simulink model "soc_dvbs2_fpga"  (R2025b)
settings: Solver=FixedStepDiscrete  StartTime=0.0  StopTime=0  RelTol=1e-3
InitFcn:
  | soc_dvbs2_init;
values from neighbouring files (symbols this model uses):
  Rsym = 4e6    (= 4000000)    [soc_dvbs2_init.m]
  soc_dvbs2_txPacketBits = [1 1 0 1 0 1 1 1 0 1 1 1 ... (2972 elements, 2972x1)]    [soc_dvbs2_txPacketBits.mat]
  syncWord = (dec2bin(hex2dec('AC')) - '0').'    [soc_dvbs2_init.m]
  txDataOut = txobj(frameBits(:))    [soc_dvbs2_init.m]
  txFiltCoeff = txobj.pTxFilterCoeff    [soc_dvbs2_init.m]
undefined symbols (not defined in the file or in its folder): Add, coefficientsLog, coefficientsSqrt1, coefficientsSqrt2, dataBits, designMultirateFIR, noisePow, NumBits1, NumBits2, seedsURNG1, seedsURNG2, Shift, Slope1, Slope2, soc_dvbs2_designFIRFilter, txDataOutS1, txDataOutS10, txDataOutS12, txDataOutS13, txDataOutS14, txDataOutS15, txDataOutS16, txDataOutS18, txDataOutS19, txDataOutS2, txDataOutS20, txDataOutS21, txDataOutS22, txDataOutS24, txDataOutS25, txDataOutS26, txDataOutS27, txDataOutS3, txDataOutS4, txDataOutS5, txDataOutS6, txDataOutS7, txDataOutS8, txDataOutS9
libraries: simulink x214, hdlsllib x211, dspsigops x22, dsphdlfiltering2 x8, dsphdlsigops2 x5, commseqgen3 x5, dsphdlmathfun2 x3, hwlogicconnlib x2, whdledac x2, commhdlcrc x2, whdlutilities x1, whdlmod x1
(part 3 of 12)

== system soc_dvbs2_fpga/DVBS2/DVBS2 TxRx/DVB-S2 HDL Receiver/Stream Recovery/BB Header CRC Check ==
  dstartIn : Inport
  dValidIn : Inport  Port=2
  bitsIn : Inport  Port=3
  hstartIn : Inport  Port=4
  hendIn : Inport  Port=5
  hvalidIn : Inport  Port=6
  Delay{,1..3,8..13,15} (11 alike) : Delay  DelayLength=1
  Delay4 : Delay  DelayLength=26
  Delay6 : Delay  DelayLength=26
  Delay7 : Delay  DelayLength=26
  Discard CRC failed Frame : Subsystem
  General CRC Syndrome Detector HDL Optimized : commhdlcrc/General CRC Syndrome Detector HDL Optimized  Polynomial=[1 1 1 0 1 0 1 0 1]  InitialState=0  DirectMethod=off  ReflectInput=off  ReflectCRCChecksum=off  FinalXORValue=0  SimulateUsing=Code generation
  dstartOut : Outport
  dvalidIn : Outport  Port=2
  dbitsOut : Outport  Port=3
  hbitsOut : Outport  Port=4
  hstartOut : Outport  Port=5
  hendOut : Outport  Port=6
  hvalidOut : Outport  Port=7
  herrorOut : Outport  Port=8
  wires:
  Delay15/1 -> Delay4/1
  dValidIn/1 -> Delay13/1
  Delay12/1 -> General CRC Syndrome Detector HDL Optimized/4
  Delay11/1 -> General CRC Syndrome Detector HDL Optimized/3
  Delay10/1 -> General CRC Syndrome Detector HDL Optimized/2
  Delay9/1 -> General CRC Syndrome Detector HDL Optimized/1, Delay7/1
  Discard CRC failed Frame/3(bitsOut) -> dbitsOut/1
  Discard CRC failed Frame/2(validOut) -> dvalidIn/1
  Discard CRC failed Frame/1(startOut) -> dstartOut/1
  Delay7/1 -> Discard CRC failed Frame/3(bitsIn)
  Delay6/1 -> Discard CRC failed Frame/2(validIn)
  Delay4/1 -> Discard CRC failed Frame/1(startIn)
  Delay8/1 -> hbitsOut/1
  Delay3/1 -> hstartOut/1
  Delay2/1 -> hendOut/1
  Delay1/1 -> hvalidOut/1
  Delay/1 -> herrorOut/1
  General CRC Syndrome Detector HDL Optimized/5 -> Delay/1, Discard CRC failed Frame/4(err)
  General CRC Syndrome Detector HDL Optimized/4 -> Delay1/1
  General CRC Syndrome Detector HDL Optimized/1 -> Delay8/1
  hvalidIn/1 -> Delay12/1
  hstartIn/1 -> Delay10/1
  bitsIn/1 -> Delay9/1
  General CRC Syndrome Detector HDL Optimized/3 -> Delay2/1, Discard CRC failed Frame/5(errorValid)
  dstartIn/1 -> Delay15/1
  Delay13/1 -> Delay6/1
  hendIn/1 -> Delay11/1
  General CRC Syndrome Detector HDL Optimized/2 -> Delay3/1

== system soc_dvbs2_fpga/DVBS2/DVBS2 TxRx/DVB-S2 HDL Receiver/Synchronizer and PL Header Decoder/Enable MODCOD  ==
  note: force MODCOD to 0 until synchronization is done
  modcod : Inport
  enb : Inport  Port=2
  Constant : Constant  Value=0  OutDataTypeStr=Inherit: Inherit via back propagation  SampleTime=-1
  Constant1 : Constant  Value=modcodToZero  OutDataTypeStr=boolean  SampleTime=-1
  Switch : Switch  Criteria=u2 ~= 0  SaturateOnIntegerOverflow=off  InputSameDT=off
  Switch1 : Switch  Criteria=u2 ~= 0  SaturateOnIntegerOverflow=off  InputSameDT=off
  modcodOut : Outport
  wires:
  modcod/1 -> Switch1/3, Switch/1
  Switch/1 -> Switch1/1
  enb/1 -> Switch/2
  Constant/1 -> Switch/3
  Constant1/1 -> Switch1/2
  Switch1/1 -> modcodOut/1

== system soc_dvbs2_fpga/DVBS2/DVBS2 TxRx/DVB-S2 HDL Receiver/Synchronizer and PL Header Decoder/Fine Phase Synchronizer ==
  dataIn : Inport
  validIn : Inport  Port=2
  endOfPLSCIn : Inport  Port=3
  mod : Inport  Port=4
  En : Inport  Port=5
  rst : Inport  Port=6
  Data Type Conversion : DataTypeConversion  OutDataTypeStr=fixdt(1,18,14)  SaturateOnIntegerOverflow=off  RndMeth=Floor
  Data Type Conversion1 : DataTypeConversion  OutDataTypeStr=fixdt(1,22,14)  SaturateOnIntegerOverflow=off  RndMeth=Floor
  Delay{1..4,12..14} (7 alike) : Delay  DelayLength=1
  Delay{5..11,15..16} (9 alike) : Delay
  Direct Digital Synthesis : Subsystem
  Loop Filter : Subsystem
  Math Function : Math  Operator=conj
  Phase Error Detector : Subsystem
  Power Q and Beta Offset Rotation : Subsystem
  Product : Product
  dataOut : Outport
  validOut : Outport  Port=2
  endOfPLSC : Outport  Port=3
  wires:
  Loop Filter/2(rstOut) -> Direct Digital Synthesis/2(rst)
  rst/1 -> Loop Filter/3(rst)
  En/1 -> Loop Filter/2(En)
  Data Type Conversion1/1 -> Delay12/1, Delay15/1
  Power Q and Beta Offset Rotation/1(dataOut) -> Phase Error Detector/1(dataIn)
  Loop Filter/1(v) -> Direct Digital Synthesis/1(v)
  Data Type Conversion/1 -> dataOut/1
  Delay16/1 -> Power Q and Beta Offset Rotation/2(mod)
  Delay15/1 -> Power Q and Beta Offset Rotation/1(dataIn)
  Delay14/1 -> endOfPLSC/1
  Delay13/1 -> validOut/1
  Delay12/1 -> Data Type Conversion/1
  Delay11/1 -> Delay14/1
  Delay10/1 -> Delay13/1
  Delay9/1 -> Delay11/1
  Delay8/1 -> Delay10/1
  Delay7/1 -> Data Type Conversion1/1
  Delay6/1 -> Product/2
  Delay5/1 -> Product/1
  endOfPLSCIn/1 -> Delay3/1
  validIn/1 -> Delay2/1
  Delay4/1 -> Delay5/1
  Delay1/1 -> Delay16/1
  Math Function/1 -> Delay6/1
  Direct Digital Synthesis/1(xph) -> Math Function/1
  Phase Error Detector/1(e) -> Loop Filter/1(e)
  mod/1 -> Delay1/1
  dataIn/1 -> Delay4/1
  Delay3/1 -> Delay9/1
  Product/1 -> Delay7/1
  Delay2/1 -> Delay8/1

== system soc_dvbs2_fpga/DVBS2/DVBS2 TxRx/DVB-S2 HDL Receiver/Synchronizer and PL Header Decoder/PL Header Recovery ==
  dataIn : Inport
  validIn : Inport  Port=2
  endOfSOF : Inport  Port=3
  hasPilots : Inport  Port=4
  Bus Creator : BusCreator  Inputs=2
  Delay{,1..3,5,11..20} (15 alike) : Delay  DelayLength=1
  Delay10 : Delay  DelayLength=46
  Delay4 : Delay  DelayLength=3
  Delay6 : Delay  DelayLength=3
  Delay7 : Delay  DelayLength=3
  Delay8 : Delay  DelayLength=46
  Delay9 : Delay  DelayLength=46
  No HDL : Subsystem
  No HDL1 : Subsystem
      settings: PortSchema="{\"entries\":[{\"content\":{\"sides\":[{\"content\":{\"connectorIds\":[\"In1\"]},\"type\":\"ConnectorPlacement.EquallySpacedRectSide\",\"uuid\":\"e49ce245-8ab6-4c67-8264-d94e0436676a\"},{\"content\":{\"connectorIds\":[\"In2\"],\"side\":\"RIGHT\"},\"type\":\"ConnectorPlacement.EquallySpacedRectSide\",\"uuid\":\"e18f2063-2732-4c7b-85c5-c61d406b5847\"},{\"content\":{\"connectorIds\":[],\"side\":\"TOP\"},\"type\":\"ConnectorPlacement.EquallySpacedRectSide\",\"uuid\":\"5432424d-e7f9-486b-a8e9-0d688bdbd9bb\"}]},\"type\":\"ConnectorPlacement.EquallySpacedConnector\",\"uuid\":\"00f6af48-98de-42b3-a1ba-3135a9ec94ea\"}],\"packageUris\":[\"http://schema.mathworks.com/mf0/Connector/R2020b\"],\"version\":\"1.0\"}"
  PL Frame Demultiplexer : Subsystem
  PL Header Decoder : Subsystem
  Unit Delay Enabled Synchronous : hdlsllib/Discrete/Unit Delay Enabled Synchronous  InitialCondition=0.0  SampleTime=-1
  Unit Delay Enabled Synchronous1 : hdlsllib/Discrete/Unit Delay Enabled Synchronous  InitialCondition=0.0  SampleTime=-1
  Unit Delay Enabled Synchronous2 : hdlsllib/Discrete/Unit Delay Enabled Synchronous  InitialCondition=0.0  SampleTime=-1
  PLSCDiag : Outport  VectorParamsAs1DForOutWhenUnconnected=off
  dataOut : Outport  Port=2  VectorParamsAs1DForOutWhenUnconnected=off
  validOut : Outport  Port=3  VectorParamsAs1DForOutWhenUnconnected=off
  endOfPLSC : Outport  Port=4  VectorParamsAs1DForOutWhenUnconnected=off
  modcod : Outport  Port=5  VectorParamsAs1DForOutWhenUnconnected=off
  FEC : Outport  Port=6  VectorParamsAs1DForOutWhenUnconnected=off
  wires:
  Unit Delay Enabled Synchronous2/1 -> FEC/1
  Unit Delay Enabled Synchronous/1 -> modcod/1
  Delay20/1 -> endOfPLSC/1
  Delay19/1 -> validOut/1
  Delay16/1 -> dataOut/1
  Bus Creator/1 -> PLSCDiag/1
  Delay18/1 -> No HDL1/2(endOfPLSc), Delay20/1, Unit Delay Enabled Synchronous/2, Unit Delay Enabled Synchronous2/2
  Delay17/1 -> Delay19/1
  Delay15/1 -> Unit Delay Enabled Synchronous2/1
  Delay14/1 -> Unit Delay Enabled Synchronous/1
  Delay13/1 -> Delay16/1
  Delay12/1 -> Delay13/1
  Delay11/1 -> Delay17/1
  Delay/1 -> Delay18/1
  Delay10/1 -> Delay12/1
  Delay9/1 -> Delay/1
  Delay8/1 -> Delay11/1
  Delay7/1 -> PL Header Decoder/3(endOfSOF)
  Delay6/1 -> PL Header Decoder/2(hasPilots)
  Delay4/1 -> Bus Creator/1, Delay10/1, PL Header Decoder/1(dataIn)  "PLSCSymb"
  Delay3/1 -> PL Frame Demultiplexer/2(validIn), No HDL1/1(valid)
  Delay2/1 -> Delay7/1, PL Frame Demultiplexer/1(endOfSOFIn), Unit Delay Enabled Synchronous1/2
  Delay1/1 -> Unit Delay Enabled Synchronous1/1
  Delay5/1 -> Delay4/1
  PL Frame Demultiplexer/3(endOfPLSC) -> Delay9/1
  PL Frame Demultiplexer/2(dValid) -> Delay8/1
  validIn/1 -> Delay3/1
  PL Frame Demultiplexer/1(hValid) -> PL Header Decoder/4(validIn), Bus Creator/2  "PLSCSymbValid"
  PL Header Decoder/2(FECFrame) -> Delay15/1
  Unit Delay Enabled Synchronous1/1 -> Delay6/1
  hasPilots/1 -> No HDL/1(has Pilots), Delay1/1
  endOfSOF/1 -> No HDL/Enable, Delay2/1
  PL Header Decoder/1(modcod) -> Delay14/1
  dataIn/1 -> Delay5/1

== system soc_dvbs2_fpga/DVBS2/DVBS2 TxRx/DVB-S2 HDL Receiver/Synchronizer and PL Header Decoder/Source Encoding ==
  modcod : Inport
  Delay1 : Delay  DelayLength=1
  Delay12 : Delay  DelayLength=1
  MATLAB Function : MATLAB Function  TreatAsAtomicUnit=on
  Terminator : Terminator
  mod : Outport
  wires:
  Delay1/1 -> mod/1
  Delay12/1 -> MATLAB Function/1(In)
  MATLAB Function/2(isdummy) -> Terminator/1
  MATLAB Function/1(out) -> Delay1/1
  modcod/1 -> Delay12/1

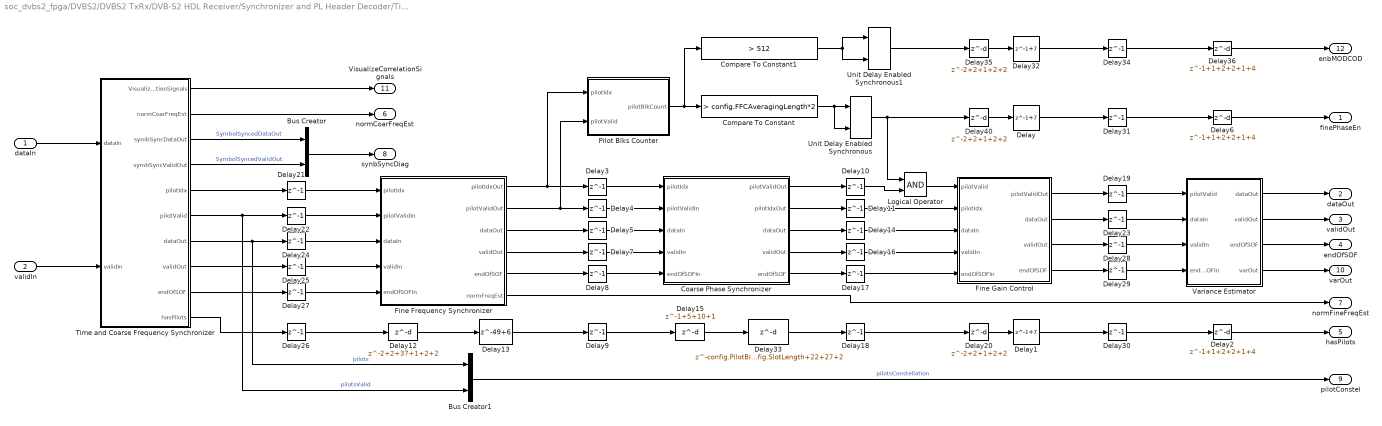
== system soc_dvbs2_fpga/DVBS2/DVBS2 TxRx/DVB-S2 HDL Receiver/Synchronizer and PL Header Decoder/Time Frequency and Coarse Phase Synchronizer ==
  dataIn : Inport
  validIn : Inport  Port=2
  Bus Creator : BusCreator  Inputs=2
  Bus Creator1 : BusCreator  Inputs=2
  Coarse Phase Synchronizer : Subsystem
  Compare To Constant : simulink/Logic and Bit Operations/Compare To Constant  relop=>  const=config.FFCAveragingLength*2  OutDataTypeStr=boolean
  Compare To Constant1 : simulink/Logic and Bit Operations/Compare To Constant  relop=>  const=512  OutDataTypeStr=boolean
  Delay : Delay  DelayLength=1+7
  Delay1 : Delay  DelayLength=1+7
  Delay{3..5,7..11,14,16..19,21..31,34} (25 alike) : Delay  DelayLength=1
  Delay12 : Delay  DelayLength=2+2+37+1+2+2
  Delay13 : Delay  DelayLength=49+6
  Delay15 : Delay  DelayLength=1+5+10+1
  Delay2 : Delay  DelayLength=1+1+2+2+1+4
  Delay20 : Delay  DelayLength=2+2+1+2+2
  Delay32 : Delay  DelayLength=1+7
  Delay33 : Delay  DelayLength=config.PilotBlkFreq*config.SlotLength+22+27+2
  Delay35 : Delay  DelayLength=2+2+1+2+2
  Delay36 : Delay  DelayLength=1+1+2+2+1+4
  Delay40 : Delay  DelayLength=2+2+1+2+2
  Delay6 : Delay  DelayLength=1+1+2+2+1+4
  Fine Frequency Synchronizer : Subsystem
  Fine Gain Control : Subsystem
  Logical Operator : Logic  AllPortsSameDT=off  OutDataTypeStr=boolean
  Pilot Blks Counter : Subsystem
  Time and Coarse Frequency Synchronizer : Subsystem
  Unit Delay Enabled Synchronous : hdlsllib/Discrete/Unit Delay Enabled Synchronous  InitialCondition=0.0  SampleTime=-1
  Unit Delay Enabled Synchronous1 : hdlsllib/Discrete/Unit Delay Enabled Synchronous  InitialCondition=0.0  SampleTime=-1
  Variance Estimator : Subsystem
  finePhaseEn : Outport
  dataOut : Outport  Port=2
  validOut : Outport  Port=3
  endOfSOF : Outport  Port=4
  hasPilots : Outport  Port=5
  normCoarFreqEst : Outport  Port=6
  normFineFreqEst : Outport  Port=7
  synbSyncDiag : Outport  Port=8
  pilotConstel : Outport  Port=9
  varOut : Outport  Port=10
  VisualizeCorrelationSignals : Outport  Port=11
  enbMODCOD : Outport  Port=12
  wires:
  Delay31/1 -> Delay6/1
  Delay30/1 -> Delay2/1
  Delay29/1 -> Variance Estimator/4(endOfSOFIn)
  Delay28/1 -> Variance Estimator/3(validIn)
  Delay23/1 -> Variance Estimator/2(dataIn)
  Delay19/1 -> Variance Estimator/1(pilotValid)
  Delay18/1 -> Delay20/1
  Delay17/1 -> Fine Gain Control/5(endOfSOFIn)
  Delay16/1 -> Fine Gain Control/4(validIn)
  Delay14/1 -> Fine Gain Control/3(dataIn)
  Delay11/1 -> Fine Gain Control/2(pilotIdx)
  Delay10/1 -> Logical Operator/2
  Delay9/1 -> Delay15/1
  Delay8/1 -> Coarse Phase Synchronizer/5(endOfSOFIn)
  Delay7/1 -> Coarse Phase Synchronizer/4(validIn)
  Delay5/1 -> Coarse Phase Synchronizer/3(dataIn)
  Delay4/1 -> Coarse Phase Synchronizer/2(pilotValidIn)
  Delay3/1 -> Coarse Phase Synchronizer/1(pilotIdx)
  Bus Creator1/1 -> pilotConstel/1  "pilotsConstellation"
  Unit Delay Enabled Synchronous/1 -> Delay40/1, Logical Operator/1
  Compare To Constant/1 -> Unit Delay Enabled Synchronous/1, Unit Delay Enabled Synchronous/2
  Logical Operator/1 -> Fine Gain Control/1(pilotValid)
  Fine Gain Control/2(dataOut) -> Delay23/1
  Coarse Phase Synchronizer/3(dataOut) -> Delay14/1
  Delay2/1 -> hasPilots/1
  Fine Gain Control/1(pilotValidOut) -> Delay19/1
  Variance Estimator/4(varOut) -> varOut/1
  Variance Estimator/3(endOfSOF) -> endOfSOF/1
  Variance Estimator/2(validOut) -> validOut/1
  Variance Estimator/1(dataOut) -> dataOut/1
  Fine Gain Control/4(endOfSOF) -> Delay29/1
  Fine Gain Control/3(validOut) -> Delay28/1
  Delay6/1 -> finePhaseEn/1
  Delay1/1 -> Delay30/1
  Delay/1 -> Delay31/1
  Fine Frequency Synchronizer/6(normFreqEst) -> normFineFreqEst/1
  Coarse Phase Synchronizer/5(endOfSOF) -> Delay17/1
  Coarse Phase Synchronizer/4(validOut) -> Delay16/1
  Coarse Phase Synchronizer/1(pilotValidOut) -> Delay10/1
  Coarse Phase Synchronizer/2(pilotIdxOut) -> Delay11/1
  Time and Coarse Frequency Synchronizer/4(symbSyncValidOut) -> Bus Creator/2  "SymbolSyncedValidOut"
  Time and Coarse Frequency Synchronizer/3(symbSyncDataOut) -> Bus Creator/1  "SymbolSyncedDataOut"
  Time and Coarse Frequency Synchronizer/10(hasPilots) -> Delay26/1
  Time and Coarse Frequency Synchronizer/9(endOfSOF) -> Delay27/1
  Time and Coarse Frequency Synchronizer/8(validOut) -> Delay25/1
  Time and Coarse Frequency Synchronizer/7(dataOut) -> Bus Creator1/1, Delay24/1  "pilots"
  Time and Coarse Frequency Synchronizer/6(pilotValid) -> Bus Creator1/2, Delay22/1  "pilotsValid"
  Time and Coarse Frequency Synchronizer/5(pilotIdx) -> Delay21/1
  Time and Coarse Frequency Synchronizer/2(normCoarFreqEst) -> normCoarFreqEst/1
  validIn/1 -> Time and Coarse Frequency Synchronizer/2(validIn)
  dataIn/1 -> Time and Coarse Frequency Synchronizer/1(dataIn)
  Delay40/1 -> Delay/1
  Pilot Blks Counter/1(pilotBlkCount) -> Compare To Constant1/1, Compare To Constant/1
  Bus Creator/1 -> synbSyncDiag/1
  Delay27/1 -> Fine Frequency Synchronizer/5(endOfSOFIn)
  Delay26/1 -> Delay12/1
  Delay25/1 -> Fine Frequency Synchronizer/4(validIn)
  Delay24/1 -> Fine Frequency Synchronizer/3(dataIn)
  Delay22/1 -> Fine Frequency Synchronizer/2(pilotValidIn)
  Delay21/1 -> Fine Frequency Synchronizer/1(pilotIdx)
  Delay20/1 -> Delay1/1
  Delay33/1 -> Delay18/1
  Delay15/1 -> Delay33/1
  Delay13/1 -> Delay9/1
  Delay12/1 -> Delay13/1
  Fine Frequency Synchronizer/5(endOfSOF) -> Delay8/1
  Fine Frequency Synchronizer/4(validOut) -> Delay7/1
  Fine Frequency Synchronizer/3(dataOut) -> Delay5/1
  Fine Frequency Synchronizer/2(pilotValidOut) -> Pilot Blks Counter/2(pilotValid), Delay4/1
  Fine Frequency Synchronizer/1(pilotIdxOut) -> Pilot Blks Counter/1(pilotIdx), Delay3/1
  Time and Coarse Frequency Synchronizer/1(VisualizeCorrelationSignals) -> VisualizeCorrelationSignals/1
  Delay35/1 -> Delay32/1
  Delay32/1 -> Delay34/1
  Delay36/1 -> enbMODCOD/1
  Delay34/1 -> Delay36/1
  Unit Delay Enabled Synchronous1/1 -> Delay35/1
  Compare To Constant1/1 -> Unit Delay Enabled Synchronous1/1, Unit Delay Enabled Synchronous1/2

== system soc_dvbs2_fpga/DVBS2/DVBS2 TxRx/LUT Based Tx/Subsystem1/Subsystem ==
  rst : Inport
  enb : Inport  Port=2
  modcodidx : Inport  Port=3
  Compare To Constant : simulink/Logic and Bit Operations/Compare To Constant  relop===  const=0  OutDataTypeStr=boolean
  Compare To Constant1 : simulink/Logic and Bit Operations/Compare To Constant  relop===  const=1  OutDataTypeStr=boolean
  Compare To Constant2 : simulink/Logic and Bit Operations/Compare To Constant  relop===  const=2  OutDataTypeStr=boolean
  Compare To Constant3 : simulink/Logic and Bit Operations/Compare To Constant  relop===  const=3  OutDataTypeStr=boolean
  Compare To Constant4 : simulink/Logic and Bit Operations/Compare To Constant  relop===  const=4  OutDataTypeStr=boolean
  Compare To Constant5 : simulink/Logic and Bit Operations/Compare To Constant  relop===  const=5  OutDataTypeStr=boolean
  Logical Operator : Logic  Operator=OR  Inputs=6  AllPortsSameDT=off  OutDataTypeStr=boolean
  Logical Operator{1..6} (6 alike) : Logic  AllPortsSameDT=off  OutDataTypeStr=boolean
  txLUT1 : Subsystem  mask{DataLUT=txDataOutS1}
      mask prompts: DataLUT "Data in LUT"
  txLUT2 : Subsystem  mask{DataLUT=txDataOutS2}
      mask prompts: DataLUT "Data in LUT"
  txLUT3 : Subsystem  mask{DataLUT=txDataOutS3}
      mask prompts: DataLUT "Data in LUT"
  txLUT4 : Subsystem  mask{DataLUT=txDataOutS4}
      mask prompts: DataLUT "Data in LUT"
  txLUT5 : Subsystem  mask{DataLUT=txDataOutS5}
      mask prompts: DataLUT "Data in LUT"
  txLUT6 : Subsystem  mask{DataLUT=txDataOutS6}
      mask prompts: DataLUT "Data in LUT"
  Out2 : Outport
  Out3 : Outport  Port=2
  Out4 : Outport  Port=3
  Out5 : Outport  Port=4
  Out6 : Outport  Port=5
  Out7 : Outport  Port=6
  Out1 : Outport  Port=7
  wires:
  rst/1 -> txLUT2/1(rst), txLUT3/1(rst), txLUT4/1(rst), txLUT5/1(rst), txLUT6/1(rst), txLUT1/1(rst)
  txLUT1/2(endOfLUT) -> Logical Operator1/1
  enb/1 -> txLUT1/2(enb), txLUT6/2(enb), txLUT5/2(enb), txLUT4/2(enb), txLUT3/2(enb), txLUT2/2(enb)
  txLUT6/1(Out1) -> Out7/1
  txLUT5/1(Out1) -> Out6/1
  txLUT2/1(Out1) -> Out3/1
  txLUT4/1(Out1) -> Out5/1
  txLUT3/1(Out1) -> Out4/1
  Logical Operator/1 -> Out1/1
  txLUT1/1(Out1) -> Out2/1
  Compare To Constant/1 -> Logical Operator1/2
  modcodidx/1 -> Compare To Constant5/1, Compare To Constant4/1, Compare To Constant3/1, Compare To Constant2/1, Compare To Constant1/1, Compare To Constant/1
  Logical Operator1/1 -> Logical Operator/1
  Logical Operator2/1 -> Logical Operator/2
  Logical Operator3/1 -> Logical Operator/3
  Logical Operator4/1 -> Logical Operator/4
  Logical Operator5/1 -> Logical Operator/5
  Logical Operator6/1 -> Logical Operator/6
  txLUT2/2(endOfLUT) -> Logical Operator2/1
  txLUT3/2(endOfLUT) -> Logical Operator3/1
  txLUT4/2(endOfLUT) -> Logical Operator4/1
  txLUT5/2(endOfLUT) -> Logical Operator5/1
  txLUT6/2(endOfLUT) -> Logical Operator6/1
  Compare To Constant1/1 -> Logical Operator2/2
  Compare To Constant2/1 -> Logical Operator3/2
  Compare To Constant3/1 -> Logical Operator4/2
  Compare To Constant4/1 -> Logical Operator5/2
  Compare To Constant5/1 -> Logical Operator6/2

== system soc_dvbs2_fpga/DVBS2/DVBS2 TxRx/LUT Based Tx/Subsystem1/Subsystem1 ==
  rst : Inport
  enb : Inport  Port=2
  modcodidx : Inport  Port=3
  Compare To Constant : simulink/Logic and Bit Operations/Compare To Constant  relop===  const=6  OutDataTypeStr=boolean
  Compare To Constant1 : simulink/Logic and Bit Operations/Compare To Constant  relop===  const=7  OutDataTypeStr=boolean
  Compare To Constant2 : simulink/Logic and Bit Operations/Compare To Constant  relop===  const=8  OutDataTypeStr=boolean
  Compare To Constant3 : simulink/Logic and Bit Operations/Compare To Constant  relop===  const=9  OutDataTypeStr=boolean
  Compare To Constant4 : simulink/Logic and Bit Operations/Compare To Constant  relop===  const=10  OutDataTypeStr=boolean
  Compare To Constant5 : simulink/Logic and Bit Operations/Compare To Constant  relop===  const=11  OutDataTypeStr=boolean
  Logical Operator : Logic  Operator=OR  Inputs=6  AllPortsSameDT=off  OutDataTypeStr=boolean
  Logical Operator{1..6} (6 alike) : Logic  AllPortsSameDT=off  OutDataTypeStr=boolean
  txLUT1 : Subsystem  mask{DataLUT=txDataOutS7}
      mask prompts: DataLUT "Data in LUT"
  txLUT2 : Subsystem  mask{DataLUT=txDataOutS8}
      mask prompts: DataLUT "Data in LUT"
  txLUT3 : Subsystem  mask{DataLUT=txDataOutS9}
      mask prompts: DataLUT "Data in LUT"
  txLUT4 : Subsystem  mask{DataLUT=txDataOutS10}
      mask prompts: DataLUT "Data in LUT"
  txLUT5 : Subsystem  mask{DataLUT=txDataOutS12}
      mask prompts: DataLUT "Data in LUT"
  txLUT6 : Subsystem  mask{DataLUT=txDataOutS13}
      mask prompts: DataLUT "Data in LUT"
  Out2 : Outport
  Out3 : Outport  Port=2
  Out4 : Outport  Port=3
  Out5 : Outport  Port=4
  Out6 : Outport  Port=5
  Out7 : Outport  Port=6
  Out1 : Outport  Port=7
  wires:
  Compare To Constant5/1 -> Logical Operator6/2
  Compare To Constant4/1 -> Logical Operator5/2
  Compare To Constant3/1 -> Logical Operator4/2
  Compare To Constant2/1 -> Logical Operator3/2
  Compare To Constant1/1 -> Logical Operator2/2
  txLUT6/2(endOfLUT) -> Logical Operator6/1
  txLUT5/2(endOfLUT) -> Logical Operator5/1
  txLUT4/2(endOfLUT) -> Logical Operator4/1
  txLUT3/2(endOfLUT) -> Logical Operator3/1
  txLUT2/2(endOfLUT) -> Logical Operator2/1
  Logical Operator6/1 -> Logical Operator/6
  Logical Operator5/1 -> Logical Operator/5
  Logical Operator4/1 -> Logical Operator/4
  Logical Operator3/1 -> Logical Operator/3
  Logical Operator2/1 -> Logical Operator/2
  Logical Operator1/1 -> Logical Operator/1
  modcodidx/1 -> Compare To Constant/1, Compare To Constant1/1, Compare To Constant2/1, Compare To Constant3/1, Compare To Constant4/1, Compare To Constant5/1
  Compare To Constant/1 -> Logical Operator1/2
  txLUT1/1(Out1) -> Out2/1
  Logical Operator/1 -> Out1/1
  txLUT3/1(Out1) -> Out4/1
  txLUT4/1(Out1) -> Out5/1
  txLUT2/1(Out1) -> Out3/1
  txLUT5/1(Out1) -> Out6/1
  txLUT6/1(Out1) -> Out7/1
  enb/1 -> txLUT2/2(enb), txLUT3/2(enb), txLUT4/2(enb), txLUT5/2(enb), txLUT6/2(enb), txLUT1/2(enb)
  txLUT1/2(endOfLUT) -> Logical Operator1/1
  rst/1 -> txLUT1/1(rst), txLUT6/1(rst), txLUT5/1(rst), txLUT4/1(rst), txLUT3/1(rst), txLUT2/1(rst)

== system soc_dvbs2_fpga/DVBS2/DVBS2 TxRx/LUT Based Tx/Subsystem1/Subsystem2 ==
  rst : Inport
  enb : Inport  Port=2
  modcodidx : Inport  Port=3
  Compare To Constant : simulink/Logic and Bit Operations/Compare To Constant  relop===  const=18  OutDataTypeStr=boolean
  Compare To Constant1 : simulink/Logic and Bit Operations/Compare To Constant  relop===  const=19  OutDataTypeStr=boolean
  Compare To Constant2 : simulink/Logic and Bit Operations/Compare To Constant  relop===  const=20  OutDataTypeStr=boolean
  Compare To Constant3 : simulink/Logic and Bit Operations/Compare To Constant  relop===  const=21  OutDataTypeStr=boolean
  Compare To Constant4 : simulink/Logic and Bit Operations/Compare To Constant  relop===  const=22  OutDataTypeStr=boolean
  Compare To Constant5 : simulink/Logic and Bit Operations/Compare To Constant  relop===  const=23  OutDataTypeStr=boolean
  Logical Operator : Logic  Operator=OR  Inputs=6  AllPortsSameDT=off  OutDataTypeStr=boolean
  Logical Operator{1..6} (6 alike) : Logic  AllPortsSameDT=off  OutDataTypeStr=boolean
  txLUT1 : Subsystem  mask{DataLUT=txDataOutS21}
      mask prompts: DataLUT "Data in LUT"
  txLUT2 : Subsystem  mask{DataLUT=txDataOutS22}
      mask prompts: DataLUT "Data in LUT"
  txLUT3 : Subsystem  mask{DataLUT=txDataOutS24}
      mask prompts: DataLUT "Data in LUT"
  txLUT4 : Subsystem  mask{DataLUT=txDataOutS25}
      mask prompts: DataLUT "Data in LUT"
  txLUT5 : Subsystem  mask{DataLUT=txDataOutS26}
      mask prompts: DataLUT "Data in LUT"
  txLUT6 : Subsystem  mask{DataLUT=txDataOutS27}
      mask prompts: DataLUT "Data in LUT"
  Out2 : Outport
  Out3 : Outport  Port=2
  Out4 : Outport  Port=3
  Out5 : Outport  Port=4
  Out6 : Outport  Port=5
  Out7 : Outport  Port=6
  Out1 : Outport  Port=7
  wires:
  Compare To Constant5/1 -> Logical Operator6/2
  Compare To Constant4/1 -> Logical Operator5/2
  Compare To Constant3/1 -> Logical Operator4/2
  Compare To Constant2/1 -> Logical Operator3/2
  Compare To Constant1/1 -> Logical Operator2/2
  txLUT6/2(endOfLUT) -> Logical Operator6/1
  txLUT5/2(endOfLUT) -> Logical Operator5/1
  txLUT4/2(endOfLUT) -> Logical Operator4/1
  txLUT3/2(endOfLUT) -> Logical Operator3/1
  txLUT2/2(endOfLUT) -> Logical Operator2/1
  Logical Operator6/1 -> Logical Operator/6
  Logical Operator5/1 -> Logical Operator/5
  Logical Operator4/1 -> Logical Operator/4
  Logical Operator3/1 -> Logical Operator/3
  Logical Operator2/1 -> Logical Operator/2
  Logical Operator1/1 -> Logical Operator/1
  modcodidx/1 -> Compare To Constant/1, Compare To Constant1/1, Compare To Constant2/1, Compare To Constant3/1, Compare To Constant4/1, Compare To Constant5/1
  Compare To Constant/1 -> Logical Operator1/2
  txLUT1/1(Out1) -> Out2/1
  Logical Operator/1 -> Out1/1
  txLUT3/1(Out1) -> Out4/1
  txLUT4/1(Out1) -> Out5/1
  txLUT2/1(Out1) -> Out3/1
  txLUT5/1(Out1) -> Out6/1
  txLUT6/1(Out1) -> Out7/1
  enb/1 -> txLUT2/2(enb), txLUT3/2(enb), txLUT4/2(enb), txLUT5/2(enb), txLUT6/2(enb), txLUT1/2(enb)
  txLUT1/2(endOfLUT) -> Logical Operator1/1
  rst/1 -> txLUT1/1(rst), txLUT6/1(rst), txLUT5/1(rst), txLUT4/1(rst), txLUT3/1(rst), txLUT2/1(rst)

== system soc_dvbs2_fpga/DVBS2/DVBS2 TxRx/LUT Based Tx/Subsystem1/Subsystem4 ==
  rst : Inport
  enb : Inport  Port=2
  modcodidx : Inport  Port=3
  Compare To Constant : simulink/Logic and Bit Operations/Compare To Constant  relop===  const=12  OutDataTypeStr=boolean
  Compare To Constant1 : simulink/Logic and Bit Operations/Compare To Constant  relop===  const=13  OutDataTypeStr=boolean
  Compare To Constant2 : simulink/Logic and Bit Operations/Compare To Constant  relop===  const=14  OutDataTypeStr=boolean
  Compare To Constant3 : simulink/Logic and Bit Operations/Compare To Constant  relop===  const=15  OutDataTypeStr=boolean
  Compare To Constant4 : simulink/Logic and Bit Operations/Compare To Constant  relop===  const=16  OutDataTypeStr=boolean
  Compare To Constant5 : simulink/Logic and Bit Operations/Compare To Constant  relop===  const=17  OutDataTypeStr=boolean
  Logical Operator : Logic  Operator=OR  Inputs=6  AllPortsSameDT=off  OutDataTypeStr=boolean
  Logical Operator{1..6} (6 alike) : Logic  AllPortsSameDT=off  OutDataTypeStr=boolean
  txLUT1 : Subsystem  mask{DataLUT=txDataOutS14}
      mask prompts: DataLUT "Data in LUT"
  txLUT2 : Subsystem  mask{DataLUT=txDataOutS15}
      mask prompts: DataLUT "Data in LUT"
  txLUT3 : Subsystem  mask{DataLUT=txDataOutS16}
      mask prompts: DataLUT "Data in LUT"
  txLUT4 : Subsystem  mask{DataLUT=txDataOutS18}
      mask prompts: DataLUT "Data in LUT"
  txLUT5 : Subsystem  mask{DataLUT=txDataOutS19}
      mask prompts: DataLUT "Data in LUT"
  txLUT6 : Subsystem  mask{DataLUT=txDataOutS20}
      mask prompts: DataLUT "Data in LUT"
  Out2 : Outport
  Out3 : Outport  Port=2
  Out4 : Outport  Port=3
  Out5 : Outport  Port=4
  Out6 : Outport  Port=5
  Out7 : Outport  Port=6
  Out1 : Outport  Port=7
  wires:
  rst/1 -> txLUT2/1(rst), txLUT3/1(rst), txLUT4/1(rst), txLUT5/1(rst), txLUT6/1(rst), txLUT1/1(rst)
  txLUT1/2(endOfLUT) -> Logical Operator1/1
  enb/1 -> txLUT1/2(enb), txLUT6/2(enb), txLUT5/2(enb), txLUT4/2(enb), txLUT3/2(enb), txLUT2/2(enb)
  txLUT6/1(Out1) -> Out7/1
  txLUT5/1(Out1) -> Out6/1
  txLUT2/1(Out1) -> Out3/1
  txLUT4/1(Out1) -> Out5/1
  txLUT3/1(Out1) -> Out4/1
  Logical Operator/1 -> Out1/1
  txLUT1/1(Out1) -> Out2/1
  Compare To Constant/1 -> Logical Operator1/2
  modcodidx/1 -> Compare To Constant5/1, Compare To Constant4/1, Compare To Constant3/1, Compare To Constant2/1, Compare To Constant1/1, Compare To Constant/1
  Logical Operator1/1 -> Logical Operator/1
  Logical Operator2/1 -> Logical Operator/2
  Logical Operator3/1 -> Logical Operator/3
  Logical Operator4/1 -> Logical Operator/4
  Logical Operator5/1 -> Logical Operator/5
  Logical Operator6/1 -> Logical Operator/6
  txLUT2/2(endOfLUT) -> Logical Operator2/1
  txLUT3/2(endOfLUT) -> Logical Operator3/1
  txLUT4/2(endOfLUT) -> Logical Operator4/1
  txLUT5/2(endOfLUT) -> Logical Operator5/1
  txLUT6/2(endOfLUT) -> Logical Operator6/1
  Compare To Constant1/1 -> Logical Operator2/2
  Compare To Constant2/1 -> Logical Operator3/2
  Compare To Constant3/1 -> Logical Operator4/2
  Compare To Constant4/1 -> Logical Operator5/2
  Compare To Constant5/1 -> Logical Operator6/2

== system soc_dvbs2_fpga/DVBS2/DVBS2 TxRx/Channel/AWGN Generator/Unit Variance Gaussian Noise/SinCos ==
  u1 : Inport
  Delay : Delay
  Delay1 : Delay
  Delay2 : Delay  DelayLength=1
  Delay3 : Delay  DelayLength=1
  Sine HDL Optimized1 : hdlsllib/Lookup Tables/Cosine HDL Optimized  OutputFormula=cos(2*pi*u)  NumDataPoints=1024  TableDataTypeStr=fixdt(0,15,15)  SimulateLUTROMDelay=off
  Sine HDL Optimized2 : hdlsllib/Lookup Tables/Cosine HDL Optimized  OutputFormula=sin(2*pi*u)  NumDataPoints=1024  TableDataTypeStr=fixdt(0,15,15)  SimulateLUTROMDelay=off
  g0 : Outport
  g1(16,15) : Outport  Port=2
  wires:
  u1/1 -> Delay2/1, Delay3/1
  Sine HDL Optimized2/1 -> Delay/1  "g0"
  Sine HDL Optimized1/1 -> Delay1/1  "g1(16,15)"
  Delay/1 -> g0/1
  Delay1/1 -> g1(16,15)/1
  Delay2/1 -> Sine HDL Optimized2/1
  Delay3/1 -> Sine HDL Optimized1/1

== system soc_dvbs2_fpga/DVBS2/DVBS2 TxRx/Channel/AWGN Generator/Unit Variance Gaussian Noise/SqrtImplementation ==
  u : Inport
  Constant : Constant  Value=0  OutDataTypeStr=fixdt(0,17,13)  SampleTime=-1
  Delay : Delay  DelayLength=19
  Delay1 : Delay  DelayLength=19
  SqrtEval : Subsystem
  Switch : Switch  Criteria=u2 ~= 0  SaturateOnIntegerOverflow=off  InputSameDT=off
  f : Outport  VectorParamsAs1DForOutWhenUnconnected=off
  wires:
  Switch/1 -> f/1
  Constant/1 -> Delay1/1
  SqrtEval/1(f) -> Switch/1
  u/1 -> SqrtEval/1(u), Delay/1
  Delay/1 -> Switch/2
  Delay1/1 -> Switch/3

== system soc_dvbs2_fpga/DVBS2/DVBS2 TxRx/Channel/AWGN Generator/Unit Variance Gaussian Noise/TausUniformRandGen ==
  ConcatandExtract : Subsystem
  TausURNG1 : Subsystem
  TausURNG2 : Subsystem
  u0(16,16) : Outport
  u1(16,16) : Outport  Port=2
  wires:
  TausURNG2/1(b) -> ConcatandExtract/2(b)  "b(32,0)"
  TausURNG1/1(a) -> ConcatandExtract/1(a)  "a(32,0)"
  ConcatandExtract/2(u1(16,16)) -> u1(16,16)/1  "u1(16,16)"
  ConcatandExtract/1(u0(48,48)) -> u0(16,16)/1  "u0(48,48)"

== system soc_dvbs2_fpga/DVBS2/DVBS2 TxRx/Channel/AWGN Generator/Unit Variance Gaussian Noise/logImplementation ==
  u0(48,48) : Inport
  Constant : Constant  Value=0  OutDataTypeStr=fixdt(0,16,9)  SampleTime=-1
  Delay : Delay  DelayLength=24
  Switch : Switch  Criteria=u2 ~= 0  SaturateOnIntegerOverflow=off  InputSameDT=off
  log : Subsystem
  e : Outport
  wires:
  Constant/1 -> Switch/3
  Switch/1 -> e/1
  log/1(e) -> Switch/1
  u0(48,48)/1 -> Delay/1, log/1(u0(48,48))
  Delay/1 -> Switch/2

== system soc_dvbs2_fpga/DVBS2/DVBS2 TxRx/DVB-S2 HDL Receiver/Demod Deinterleave and FECDecode/DVBS2 HDL Deinterleaver/RAM ==
  wr_din : Inport
  wr_addr : Inport  Port=2
  wr_en : Inport  Port=3
  rd_addr : Inport  Port=4
  rd_valid : Inport  Port=5
  rd_end : Inport  Port=6
  rd_start : Inport  Port=7
  Delay : Delay  DelayLength=1
  Delay1 : Delay  DelayLength=1
  Delay{3..13} (11 alike) : Delay
  Delay2 : Delay  DelayLength=1
  Single RAM Using Two RAMs : Subsystem
  Wrap Address : Subsystem
  rd_dout : Outport
  rd_startOut : Outport  Port=2
  rd_endOut : Outport  Port=3
  rd_validOut : Outport  Port=4
  wires:
  Delay13/1 -> rd_endOut/1
  Delay11/1 -> rd_startOut/1
  Delay10/1 -> rd_validOut/1
  Delay9/1 -> rd_dout/1
  Delay5/1 -> Delay2/1
  Delay4/1 -> Delay1/1
  Delay3/1 -> Delay/1
  Wrap Address/1(y) -> Delay8/1
  rd_addr/1 -> Wrap Address/1(u)
  Delay2/1 -> Delay13/1
  Delay1/1 -> Delay11/1
  rd_end/1 -> Delay5/1
  rd_start/1 -> Delay4/1
  Delay/1 -> Delay10/1
  rd_valid/1 -> Delay3/1
  wr_addr/1 -> Delay6/1
  wr_din/1 -> Delay12/1
  wr_en/1 -> Delay7/1
  Delay12/1 -> Single RAM Using Two RAMs/1(wr_din)
  Delay6/1 -> Single RAM Using Two RAMs/2(wr_addr)
  Delay7/1 -> Single RAM Using Two RAMs/3(wr_en)
  Delay8/1 -> Single RAM Using Two RAMs/4(rd_addr)
  Single RAM Using Two RAMs/1(rd_dout) -> Delay9/1

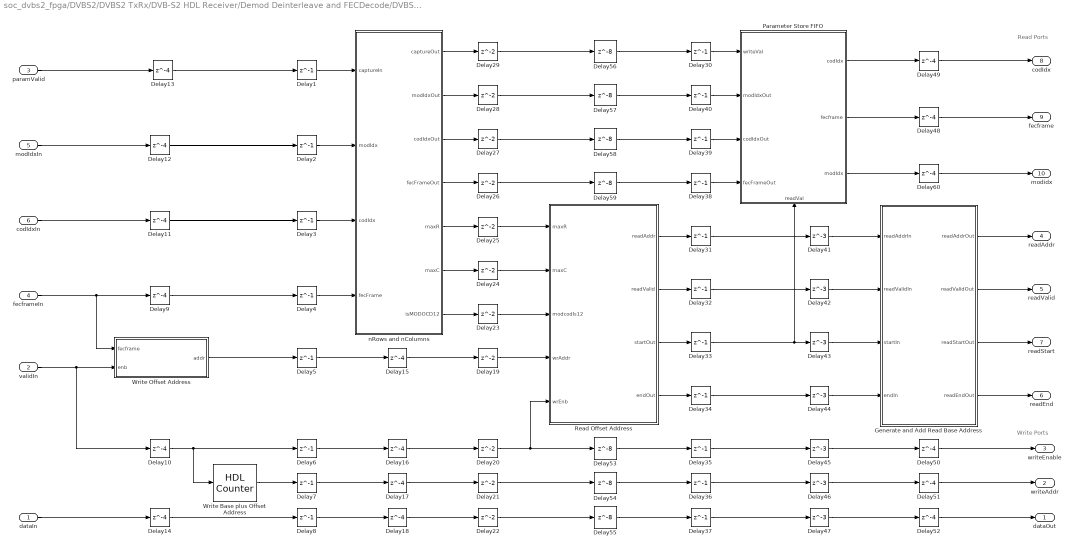
== system soc_dvbs2_fpga/DVBS2/DVBS2 TxRx/DVB-S2 HDL Receiver/Demod Deinterleave and FECDecode/DVBS2 HDL Deinterleaver/RAM Address Generator ==
  note: Write Ports
  note: Read Ports
  dataIn : Inport
  validIn : Inport  Port=2
  paramValid : Inport  Port=3
  fecframeIn : Inport  Port=4
  modIdxIn : Inport  Port=5
  codIdxIn : Inport  Port=6
  Delay{1..8,30..40} (19 alike) : Delay  DelayLength=1
  Delay{9..18,48..52,60} (16 alike) : Delay  DelayLength=4
  Delay{19..29} (11 alike) : Delay
  Delay{41..47} (7 alike) : Delay  DelayLength=3
  Delay{53..59} (7 alike) : Delay  DelayLength=8
  Generate and Add Read Base Address : Subsystem
  Parameter Store FIFO : Subsystem
      settings: PortSchema="{\"entries\":[{\"content\":{\"sides\":[{\"content\":{\"connectorIds\":[\"In1\",\"In2\",\"In3\",\"In4\"]},\"type\":\"ConnectorPlacement.EquallySpacedRectSide\",\"uuid\":\"6d8768ca-7228-4729-bdbf-9ebbcab1a5aa\"},{\"content\":{\"connectorIds\":[\"Out1\",\"Out2\",\"Out3\"],\"side\":\"RIGHT\"},\"type\":\"ConnectorPlacement.EquallySpacedRectSide\",\"uuid\":\"b8ba0d5a-2b82-4d8d-a9c2-2d3fcacc6c9a\"},{\"content\":{\"connectorIds\":[],\"side\":\"TOP\"},\"type\":\"ConnectorPlacement.EquallySpacedRectSide\",\"uuid\":\"1722486f-4cf2-41b6-8f78-86c27924cee8\"},{\"content\":{\"connectorIds\":[\"In5\"],\"side\":\"BOTTOM\"},\"type\":\"ConnectorPlacement.EquallySpacedRectSide\",\"uuid\":\"409cf5cf-743f-45fc-b63a-6af4afdbc038\"}]},\"type\":\"ConnectorPlacement.EquallySpacedConnector\",\"uuid\":\"90aa5513-49d5-48a8-89f8-bb5993d63f9c\"}],\"packageUris\":[\"http://schema.mathworks.com/mf0/Connector/R2020b\"],\"version\":\"1.0\"}"
  Read Offset Address : Subsystem
  Write Base plus Offset Address : hdlsllib/Sources/HDL Counter  CountType=Count limited  CountInit=0  CountStep=1  CountMax=ConfigRx.RAMCapacity - 1  CountFromType=Initial value  CountFrom=0  CountResetPort=off  CountLoadPort=off  CountEnbPort=on  CountDirPort=off  CountHitOutputPort=off  CountDataType=Unsigned  CountWordLen=nextpow2(ConfigRx.RAMCapacity - 1)  CountFracLen=0  CountSampTime=1
  Write Offset Address : Subsystem
  nRows and nColumns : Subsystem
  dataOut : Outport
  writeAddr : Outport  Port=2
  writeEnable : Outport  Port=3
  readAddr : Outport  Port=4
  readValid : Outport  Port=5
  readEnd : Outport  Port=6
  readStart : Outport  Port=7
  codIdx : Outport  Port=8
  fecframe : Outport  Port=9
  modidx : Outport  Port=10
  wires:
  Read Offset Address/4(endOut) -> Delay34/1
  Read Offset Address/3(startOut) -> Delay33/1
  Read Offset Address/2(readValid) -> Delay32/1
  Read Offset Address/1(readAddr) -> Delay31/1
  Delay19/1 -> Read Offset Address/4(wrAddr)
  Delay23/1 -> Read Offset Address/3(modcodIs12)
  Delay24/1 -> Read Offset Address/2(maxC)
  Delay25/1 -> Read Offset Address/1(maxR)
  Delay56/1 -> Delay30/1
  Delay57/1 -> Delay40/1
  Delay58/1 -> Delay39/1
  Delay59/1 -> Delay38/1
  Delay55/1 -> Delay37/1
  Delay54/1 -> Delay36/1
  Delay53/1 -> Delay35/1
  Delay52/1 -> dataOut/1
  Delay51/1 -> writeAddr/1
  Delay50/1 -> writeEnable/1
  Delay49/1 -> codIdx/1
  Delay48/1 -> fecframe/1
  Delay47/1 -> Delay52/1
  Delay46/1 -> Delay51/1
  Delay45/1 -> Delay50/1
  Delay44/1 -> Generate and Add Read Base Address/4(endIn)
  Delay43/1 -> Generate and Add Read Base Address/3(startIn)
  Delay42/1 -> Generate and Add Read Base Address/2(readValidIn)
  Delay41/1 -> Generate and Add Read Base Address/1(readAddrIn)
  Delay40/1 -> Parameter Store FIFO/2(modIdxOut)
  Delay39/1 -> Parameter Store FIFO/3(codIdxOut)
  Delay38/1 -> Parameter Store FIFO/4(fecFrameOut)
  Delay37/1 -> Delay47/1
  Delay36/1 -> Delay46/1
  Delay35/1 -> Delay45/1
  Delay34/1 -> Delay44/1
  Delay33/1 -> Parameter Store FIFO/5(readVal), Delay43/1
  Delay32/1 -> Delay42/1
  Delay31/1 -> Delay41/1
  Delay30/1 -> Parameter Store FIFO/1(writeVal)
  Delay29/1 -> Delay56/1
  Delay28/1 -> Delay57/1
  Delay27/1 -> Delay58/1
  Delay26/1 -> Delay59/1
  Delay22/1 -> Delay55/1
  Delay21/1 -> Delay54/1
  Delay20/1 -> Read Offset Address/5(wrEnb), Delay53/1
  Delay18/1 -> Delay22/1
  Delay17/1 -> Delay21/1
  Delay16/1 -> Delay20/1
  Delay15/1 -> Delay19/1
  Delay1/1 -> nRows and nColumns/1(captureIn)
  Delay13/1 -> Delay1/1
  Delay14/1 -> Delay8/1
  Delay8/1 -> Delay18/1
  Delay12/1 -> Delay2/1
  Delay11/1 -> Delay3/1
  Delay10/1 -> Delay6/1, Write Base plus Offset Address/1
  Delay9/1 -> Delay4/1
  Delay7/1 -> Delay17/1
  Delay6/1 -> Delay16/1
  Delay5/1 -> Delay15/1
  Delay4/1 -> nRows and nColumns/4(fecFrame)
  Delay3/1 -> nRows and nColumns/3(codIdx)
  Delay2/1 -> nRows and nColumns/2(modIdx)
  nRows and nColumns/2(modIdxOut) -> Delay28/1
  Parameter Store FIFO/2(fecframe) -> Delay48/1
  Parameter Store FIFO/1(codIdx) -> Delay49/1
  nRows and nColumns/1(captureOut) -> Delay29/1
  nRows and nColumns/4(fecFrameOut) -> Delay26/1
  nRows and nColumns/3(codIdxOut) -> Delay27/1
  Write Offset Address/1(addr) -> Delay5/1
  Generate and Add Read Base Address/4(readEndOut) -> readEnd/1
  Generate and Add Read Base Address/3(readStartOut) -> readStart/1
  Generate and Add Read Base Address/2(readValidOut) -> readValid/1
  Generate and Add Read Base Address/1(readAddrOut) -> readAddr/1
  dataIn/1 -> Delay14/1
  codIdxIn/1 -> Delay11/1
  nRows and nColumns/7(isMODOCD12) -> Delay23/1
  fecframeIn/1 -> Write Offset Address/1(fecframe), Delay9/1
  modIdxIn/1 -> Delay12/1
  Write Base plus Offset Address/1 -> Delay7/1
  nRows and nColumns/6(maxC) -> Delay24/1
  validIn/1 -> Delay10/1, Write Offset Address/2(enb)
  nRows and nColumns/5(maxR) -> Delay25/1
  Parameter Store FIFO/3(modIdx) -> Delay60/1
  Delay60/1 -> modidx/1
  paramValid/1 -> Delay13/1

== system soc_dvbs2_fpga/DVBS2/DVBS2 TxRx/DVB-S2 HDL Receiver/Stream Recovery/BB Decoder/Extract BBHeader ==
  bitsIn : Inport
  reset : Inport  Port=2
  validIn : Inport  Port=3
  Bit Index : hdlsllib/Sources/HDL Counter  CountType=Count limited  CountInit=0  CountStep=1  CountMax=80 - 8 - 1  CountFromType=Initial value  CountFrom=0  CountResetPort=on  CountLoadPort=off  CountEnbPort=on  CountDirPort=off  CountHitOutputPort=off  CountDataType=Unsigned  CountWordLen=nextpow2(80 - 8 - 1)  CountFracLen=0  CountSampTime=1
  Extract DFL : Subsystem
  Extract MATYPE1 : Subsystem
  Extract MATYPE2 : Subsystem
  Extract SYNC : Subsystem
  Extract SYNCD : Subsystem
  Extract UPL : Subsystem
  Saturate UPL value : Subsystem
  TSorGS : Outport
  SISorMIS : Outport  Port=2
  CCMorACM : Outport  Port=3
  ISSYI : Outport  Port=4
  NPD : Outport  Port=5
  RO : Outport  Port=6
  MIS_ISI : Outport  Port=7
  UPL : Outport  Port=8
  DFL : Outport  Port=9
  SYNC : Outport  Port=10
  SYNCD : Outport  Port=11
  wires:
  Extract SYNCD/1(DFL) -> SYNCD/1
  Extract SYNC/1(SYNC) -> SYNC/1
  Extract DFL/1(DFL) -> Saturate UPL value/2(DFL), DFL/1
  Extract MATYPE2/1(MIS_ISI) -> MIS_ISI/1
  Extract MATYPE1/6(RO) -> RO/1
  Extract MATYPE1/5(NPD) -> NPD/1
  Extract MATYPE1/4(ISSYI) -> ISSYI/1
  Extract MATYPE1/3(CCMorACM) -> CCMorACM/1
  Extract MATYPE1/2(SISorMIS) -> SISorMIS/1
  Extract MATYPE1/1(TSorGS) -> TSorGS/1
  bitsIn/1 -> Extract MATYPE2/1(bitsIn), Extract UPL/1(bitsIn), Extract DFL/1(bitsIn), Extract SYNC/1(bitsIn), Extract SYNCD/1(bitsIn), Extract MATYPE1/1(bitsIn)
  validIn/1 -> Extract MATYPE1/3(validIn), Extract MATYPE2/3(validIn), Extract UPL/3(validIn), Extract DFL/3(validIn), Extract SYNC/3(validIn), Extract SYNCD/3(validIn), Bit Index/2
  reset/1 -> Bit Index/1
  Bit Index/1 -> Extract MATYPE1/2(idx), Extract MATYPE2/2(idx), Extract UPL/2(idx), Extract DFL/2(idx), Extract SYNCD/2(idx), Extract SYNC/2(idx)
  Extract UPL/1(UPL) -> Saturate UPL value/1(UPL)
  Saturate UPL value/1(saturatedUPL) -> UPL/1

== system soc_dvbs2_fpga/DVBS2/DVBS2 TxRx/DVB-S2 HDL Receiver/Stream Recovery/BB Decoder/Extract Data Field ==
  dataIn : Inport
  startIn : Inport  Port=2
  validIn : Inport  Port=3
  DFL : Inport  Port=4
  Delay{2,19..21} (4 alike) : Delay  DelayLength=1
  Indicate SYNCD bit : Subsystem
  Sample Discard Control : MATLAB Function  TreatAsAtomicUnit=on
  dataOut : Outport
  startOut : Outport  Port=2
  endOut : Outport  Port=3
  validOut : Outport  Port=4
  wires:
  Indicate SYNCD bit/1(trigger) -> Sample Discard Control/3(endIn)
  DFL/1 -> Delay2/1
  dataIn/1 -> Delay19/1
  validIn/1 -> Delay21/1
  Delay21/1 -> Indicate SYNCD bit/3(validIn), Sample Discard Control/4(validIn)
  Delay2/1 -> Indicate SYNCD bit/2(Distance)
  Delay20/1 -> Sample Discard Control/2(startIn)
  Delay19/1 -> Sample Discard Control/1(dataIn)
  startIn/1 -> Indicate SYNCD bit/1(rst), Delay20/1
  Sample Discard Control/1(dataOut) -> dataOut/1
  Sample Discard Control/2(startOut) -> startOut/1
  Sample Discard Control/3(endOut) -> endOut/1
  Sample Discard Control/4(validOut) -> validOut/1

== system soc_dvbs2_fpga/DVBS2/DVBS2 TxRx/DVB-S2 HDL Receiver/Stream Recovery/BB Decoder/Extract Stream ==
  bitsIn : Inport
  startIn : Inport  Port=2
  endIn : Inport  Port=3
  validIn : Inport  Port=4
  UPL : Inport  Port=5
  SYNC : Inport  Port=6
  SYNCD : Inport  Port=7
  Constant : Constant  Value=0  OutDataTypeStr=Inherit: Inherit via back propagation  SampleTime=-1
  Constant1 : Constant  Value=0  OutDataTypeStr=Inherit: Inherit via back propagation  SampleTime=-1
  Data Type Duplicate : DataTypeDuplicate
  Delay{,1..4,11} (6 alike) : Delay  DelayLength=3
  Delay10 : Delay  DelayLength=26-8
  Delay{5..9,12} (6 alike) : Delay  DelayLength=26
  Delay{13..17} (5 alike) : Delay
  "Extract User Packet " : Subsystem
      settings: PortSchema="{\"entries\":[{\"content\":{\"sides\":[{\"content\":{\"connectorIds\":[\"In1\",\"In2\",\"In3\",\"In4\",\"In5\",\"In6\"]},\"type\":\"ConnectorPlacement.EquallySpacedRectSide\",\"uuid\":\"30bbefc6-865c-4d46-8d30-c0dc2033b40d\"},{\"content\":{\"connectorIds\":[\"Out1\",\"Out2\",\"Out3\",\"Out4\"],\"side\":\"RIGHT\"},\"type\":\"ConnectorPlacement.EquallySpacedRectSide\",\"uuid\":\"4bb8f2ab-53ab-44a5-b9cc-3263965c7c56\"},{\"content\":{\"connectorIds\":[\"Out5\"],\"side\":\"TOP\"},\"type\":\"ConnectorPlacement.EquallySpacedRectSide\",\"uuid\":\"6ba78414-1160-4c06-babf-b4f0e9c66709\"}]},\"type\":\"ConnectorPlacement.EquallySpacedConnector\",\"uuid\":\"de23a90d-3c91-48eb-9a27-8b4a67963b0a\"}],\"packageUris\":[\"http://schema.mathworks.com/mf0/Connector/R2020b\"],\"version\":\"1.0\"}"
  Insert SYNC : Subsystem
      settings: PortSchema="{\"entries\":[{\"content\":{\"sides\":[{\"content\":{\"connectorIds\":[\"In1\",\"In2\",\"In3\",\"In4\",\"In5\",\"In6\"]},\"type\":\"ConnectorPlacement.EquallySpacedRectSide\",\"uuid\":\"4cd8a141-a868-4253-b032-d3282f125cfe\"},{\"content\":{\"connectorIds\":[\"Out1\",\"Out2\",\"Out3\",\"Out4\",\"Out5\",\"Out6\"],\"side\":\"RIGHT\"},\"type\":\"ConnectorPlacement.EquallySpacedRectSide\",\"uuid\":\"7d9766a1-2532-4c70-9d0d-5fc3901c37c9\"},{\"content\":{\"connectorIds\":[\"In7\"],\"side\":\"TOP\"},\"type\":\"ConnectorPlacement.EquallySpacedRectSide\",\"uuid\":\"e7cd0309-f074-468c-ba34-988e1448b4a3\"}]},\"type\":\"ConnectorPlacement.EquallySpacedConnector\",\"uuid\":\"3096112b-1522-4a01-b20c-4a93e2859660\"}],\"packageUris\":[\"http://schema.mathworks.com/mf0/Connector/R2020b\"],\"version\":\"1.0\"}"
  Switch{,1..5} (6 alike) : Switch  Criteria=u2 ~= 0  SaturateOnIntegerOverflow=off  InputSameDT=off
  User Packet CRC Check : commhdlcrc/General CRC Syndrome Detector HDL Optimized  Polynomial=[1 1 1 0 1 0 1 0 1]  InitialState=0  DirectMethod=off  ReflectInput=off  ReflectCRCChecksum=off  FinalXORValue=0  SimulateUsing=Code generation
  bitsOut : Outport
  startOut : Outport  Port=2
  endOut : Outport  Port=3
  validOut : Outport  Port=4
  pktErr : Outport  Port=5
  invalidPkt : Outport  Port=6
  frameStart : Outport  Port=7
  frameEnd : Outport  Port=8
  wires:
  Insert SYNC/3(startOut) -> Switch1/1
  Insert SYNC/4(endOut) -> Switch2/1
  Insert SYNC/5(validOut) -> Switch3/1
  Insert SYNC/6(errOut) -> Switch4/1
  Insert SYNC/2(dataOut) -> Switch/1
  Delay9/1 -> Delay17/1
  Delay8/1 -> Delay16/1
  Delay7/1 -> Delay15/1
  Delay6/1 -> Delay14/1
  Delay5/1 -> Delay13/1
  Delay4/1 -> Delay9/1
  Delay3/1 -> Delay8/1
  Delay2/1 -> Delay7/1
  Delay1/1 -> Delay6/1
  Delay/1 -> Delay5/1
  Switch1/1 -> startOut/1
  Switch2/1 -> endOut/1
  Switch3/1 -> validOut/1
  Switch4/1 -> pktErr/1
  Constant/1 -> Switch4/3
  Switch/1 -> bitsOut/1
  bitsIn/1 -> Delay/1, "Extract User Packet "/2(bitsIn)
  validIn/1 -> Delay3/1, "Extract User Packet "/5(validIn)
  UPL/1 -> "Extract User Packet "/6(UPL), Delay4/1
  SYNCD/1 -> "Extract User Packet "/1(SYNCD)
  startIn/1 -> Delay1/1, "Extract User Packet "/3(startIn)
  "Extract User Packet "/3(endOut) -> User Packet CRC Check/3
  "Extract User Packet "/4(validOut) -> User Packet CRC Check/4
  "Extract User Packet "/2(startOut) -> User Packet CRC Check/2
  endIn/1 -> Delay2/1, "Extract User Packet "/4(endIn)
  "Extract User Packet "/1(dataOut) -> User Packet CRC Check/1
  "Extract User Packet "/5(invalidPkt) -> Delay10/1
  Insert SYNC/1(invalidOut) -> Switch5/1, Data Type Duplicate/1
  User Packet CRC Check/1 -> Insert SYNC/2(dataIn)
  User Packet CRC Check/2 -> Insert SYNC/3(startIn)
  User Packet CRC Check/3 -> Insert SYNC/4(endIn)
  User Packet CRC Check/4 -> Insert SYNC/5(validIn)
  User Packet CRC Check/5 -> Insert SYNC/6(errIn)
  Delay10/1 -> Insert SYNC/1(invalidIn)
  SYNC/1 -> Delay11/1
  Delay11/1 -> Delay12/1
  Delay12/1 -> Insert SYNC/7(SYNC)
  Delay13/1 -> Switch/3
  Delay14/1 -> frameStart/1, Switch1/3
  Delay15/1 -> frameEnd/1, Switch2/3
  Delay16/1 -> Switch3/3
  Delay17/1 -> Switch4/2, Switch3/2, Switch2/2, Switch1/2, Switch5/2, Switch/2
  Switch5/1 -> invalidPkt/1
  Constant1/1 -> Data Type Duplicate/2, Switch5/3

== system soc_dvbs2_fpga/DVBS2/DVBS2 TxRx/DVB-S2 HDL Receiver/Stream Recovery/BB Descrambler/Subsystem ==
  In1 : Inport
  Enable : EnablePort
  PN Sequence Generator : commseqgen3/PN Sequence Generator  poly='z^15 + z + 1'  ini_sta=[1 0 0 1 0 1 0 1 0 0 0 0 0 0 0]  outBitMaskSource=Dialog parameter  shift=15  outVarSiz=off  maxOutSizeMode=Dialog parameter  maxOutSize=[10 1]  Ts=-1  sampPerFrame=1  reset=on  bitPackedOutputs=off  outDataType=Smallest unsigned integer  numPackedBits=8  bitPackDataSigned=off  bitPackedOutDType=double
  Out1 : Outport  InitialOutput=0
  wires:
  In1/1 -> PN Sequence Generator/1
  PN Sequence Generator/1 -> Out1/1

== system soc_dvbs2_fpga/DVBS2/DVBS2 TxRx/DVB-S2 HDL Receiver/Stream Recovery/BB Header CRC Check/Discard CRC failed Frame ==
  startIn : Inport
  validIn : Inport  Port=2
  bitsIn : Inport  Port=3
  err : Inport  Port=4
  errorValid : Inport  Port=5
  Delay10 : Delay  DelayLength=1
  Delay12 : Delay  DelayLength=1
  Delay9 : Delay  DelayLength=1
  Logical Operator : Logic  Operator=NOT  AllPortsSameDT=off  OutDataTypeStr=boolean
  Logical Operator1 : Logic  AllPortsSameDT=off  OutDataTypeStr=boolean
  Logical Operator2 : Logic  AllPortsSameDT=off  OutDataTypeStr=boolean
  Logical Operator4 : Logic  AllPortsSameDT=off  OutDataTypeStr=boolean
  Unit Delay Enabled Resettable Synchronous : hdlsllib/Discrete/Unit Delay Enabled Resettable Synchronous  InitialCondition=0.0  SampleTime=-1
  startOut : Outport
  validOut : Outport  Port=2
  bitsOut : Outport  Port=3
  wires:
  Logical Operator4/1 -> startOut/1
  Delay12/1 -> Logical Operator4/1
  Delay10/1 -> Logical Operator2/1
  Logical Operator2/1 -> validOut/1
  Unit Delay Enabled Resettable Synchronous/1 -> Logical Operator1/2, Logical Operator4/2, Logical Operator2/2
  Delay9/1 -> Logical Operator1/1
  Logical Operator1/1 -> bitsOut/1
  Logical Operator/1 -> Unit Delay Enabled Resettable Synchronous/1
  err/1 -> Logical Operator/1, Unit Delay Enabled Resettable Synchronous/3
  errorValid/1 -> Unit Delay Enabled Resettable Synchronous/2
  bitsIn/1 -> Delay9/1
  startIn/1 -> Delay12/1
  validIn/1 -> Delay10/1
